simulink model "untitled"  (Simulink 7.6)
settings: Solver=ode45  StartTime=0.0  StopTime=inf  RelTol=1e-3
libraries: opclib x5, simulink x2
settings Model: Creator=Administrator  LastModifiedBy=Administrator

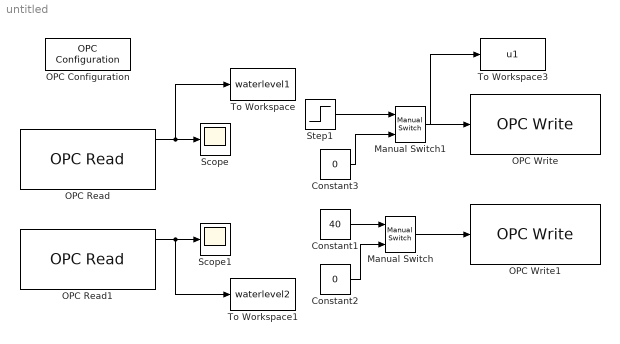
== system untitled ==
  Constant1 : Constant  Value=40
  Constant2 : Constant  Value=0
  Constant3 : Constant  Value=0
  Manual Switch : simulink/Signal Routing/Manual Switch  SystemSampleTime=-1  sw=0  action=0  varsize=off
  Manual Switch1 : simulink/Signal Routing/Manual Switch  SystemSampleTime=-1  sw=0  action=0  varsize=off
  OPC Configuration : opclib/OPC Configuration  opcServers=localhost/OPCServer.WinCC/10  errMissingItems=Error  errReadWrite=Warn  errShutdown=Error  errRTViolation=Warn  rtEnable=on  speedup=1  showLatency=off  beingUsed=on
  OPC Read : opclib/OPC Read  serverHost=localhost  serverID=OPCServer.WinCC  itemIDs=shuiwei1  readMode=Synchronous (cache)  dataType=double  updateRate=0.5  showQual=on  showTS=on  tsMode=Seconds since start
  OPC Read1 : opclib/OPC Read  serverHost=localhost  serverID=OPCServer.WinCC  itemIDs=shuiwei2  readMode=Synchronous (cache)  dataType=double  updateRate=0.5  showQual=on  showTS=on  tsMode=Seconds since start
  OPC Write : opclib/OPC Write  serverHost=localhost  serverID=OPCServer.WinCC  itemIDs=beng1  writeMode=Synchronous  updateRate=0
  OPC Write1 : opclib/OPC Write  serverHost=localhost  serverID=OPCServer.WinCC  itemIDs=beng2  writeMode=Synchronous  updateRate=0
  Scope : Scope
      settings: TimeRange=100  YMin=0  YMax=30
  Scope1 : Scope
      settings: TimeRange=100  YMin=0  YMax=30
  Step1 : Step  Time=600  Before=40  After=50
  To Workspace : ToWorkspace  VariableName=waterlevel1  SampleTime=1  SaveFormat=Array
  To Workspace1 : ToWorkspace  VariableName=waterlevel2  SampleTime=1  SaveFormat=Array
  To Workspace3 : ToWorkspace  VariableName=u1  SampleTime=1  SaveFormat=Array
  wires:
  OPC Read/1 -> Scope/1, To Workspace/1
  OPC Read1/1 -> Scope1/1, To Workspace1/1
  Constant1/1 -> Manual Switch/1
  Manual Switch/1 -> OPC Write1/1
  Constant2/1 -> Manual Switch/2
  Step1/1 -> Manual Switch1/1
  Manual Switch1/1 -> OPC Write/1, To Workspace3/1
  Constant3/1 -> Manual Switch1/2
